simulink subsystem "Inputs_ESP32"  (R2023b)
settings: Solver=VariableStepAuto  StartTime=0.0  StopTime=10.0  RelTol=1e-3
libraries: arduinolib x3
settings Model: Creator=m4ttn  LastModifiedBy=m4ttn
settings RTWCC: GPUComputeCapability=5.0

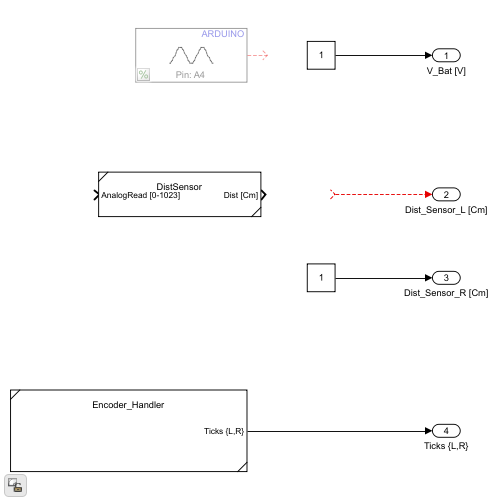
[thumbnail: Simulink's stored preview of the top-level diagram]
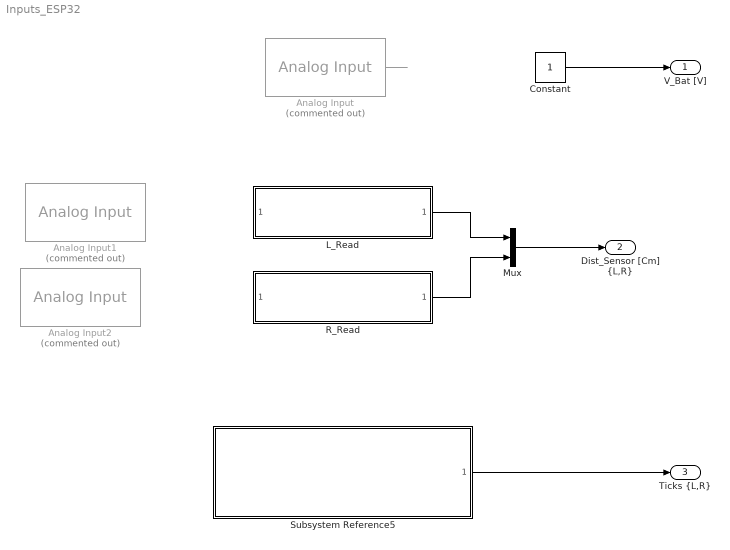
== system Inputs_ESP32 ==
  Analog Input : arduinolib/Analog Input  Commented=on  pinNumber=4  ReadResultsOnly=off  ConversionTriggerSource=Software  ExternalTriggerType=uint32( 0 )  OutputDataType=uint16  EnableConversionCompleteNotify=off  EnableOuputStatus=off  SampleTime=-1  blockPlatform=arduino
  Analog Input1 : arduinolib/Analog Input  Commented=on  pinNumber=6  ReadResultsOnly=off  ConversionTriggerSource=Software  ExternalTriggerType=uint32( 0 )  OutputDataType=uint16  EnableConversionCompleteNotify=off  EnableOuputStatus=off  SampleTime=-1  blockPlatform=arduino
  Analog Input2 : arduinolib/Analog Input  Commented=on  pinNumber=7  ReadResultsOnly=off  ConversionTriggerSource=Software  ExternalTriggerType=uint32( 0 )  OutputDataType=uint16  EnableConversionCompleteNotify=off  EnableOuputStatus=off  SampleTime=-1  blockPlatform=arduino
  Constant : Constant  OutDataTypeStr=uint16
  L_Read : Subsystem  ReferencedSubsystem=DistSensor
  Mux : Mux  Inputs=2
  R_Read : Subsystem  ReferencedSubsystem=DistSensor
  Subsystem Reference5 : Subsystem  ReferencedSubsystem=Encoder_Handler
  V_Bat [V] : Outport
  "Dist_Sensor [Cm] {L,R}" : Outport  Port=2
  "Ticks {L,R}" : Outport  Port=3
  wires:
  Analog Input/1 -> ?
  Constant/1 -> V_Bat [V]/1
  Mux/1 -> "Dist_Sensor [Cm] {L,R}"/1
  Subsystem Reference5/1 -> "Ticks {L,R}"/1
  L_Read/1 -> Mux/1
  R_Read/1 -> Mux/2
